simulink model "PIDSCF"  (Simulink 8.3)
settings: Solver=ode4  SolverMode=SingleTasking  StartTime=0.0  StopTime=10  FixedStep=0.001  RelTol=1e-3
libraries: simulink_need_slupdate x1
settings Model: Creator=Zhu Supeng  LastModifiedBy=sony
settings DataIOCC: SignalLoggingName=sigsOut
settings DebuggingCC: SaveWithParameterizedLinksMsg=none  SignalResolutionControl=TryResolveAllWithWarning  SolverPrmCheckMsg=none  MultiTaskDSMMsg=warning  MultiTaskCondExecSysMsg=none  StateNameClashWarn=none
settings HardwareCC: TargetUnknown=on
settings RTWCC: IncludeERTFirstTime=on

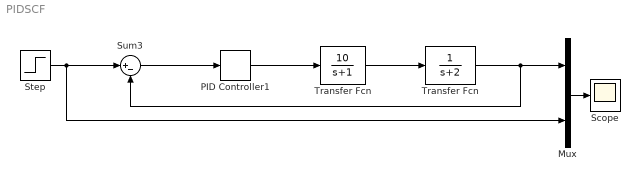
== system PIDSCF ==
  " Transfer Fcn" : TransferFcn  Denominator=[1 2]
  Mux : Mux  Inputs=2
  PID Controller1 : simulink_need_slupdate/PID Controller  P=4  I=0  D=0
  Scope : Scope
      settings: YMin=0  YMax=1.6  SaveName=PIDtu_34  MaxDataPoints=50000
  Step : Step  Time=0  SampleTime=0
  Sum3 : Sum  Inputs=|+-  SaturateOnIntegerOverflow=on
  "Transfer Fcn  " : TransferFcn  Numerator=[10]  Denominator=[1 1]
  wires:
  "Transfer Fcn  "/1 -> " Transfer Fcn"/1
  PID Controller1/1 -> "Transfer Fcn  "/1
  " Transfer Fcn"/1 -> Sum3/2, Mux/1
  Sum3/1 -> PID Controller1/1
  Mux/1 -> Scope/1
  Step/1 -> Mux/2, Sum3/1
